simulink model "non_linear_control"  (R2024b)
settings: Solver=FixedStepAuto  StartTime=0.0  StopTime=30  FixedStep=0.01  RelTol=1e-3
settings Model: Creator=olive  LastModifiedBy=olive

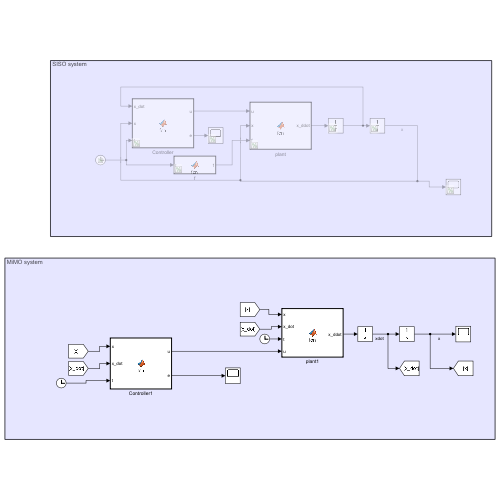
[thumbnail: Simulink's stored preview of the top-level diagram]
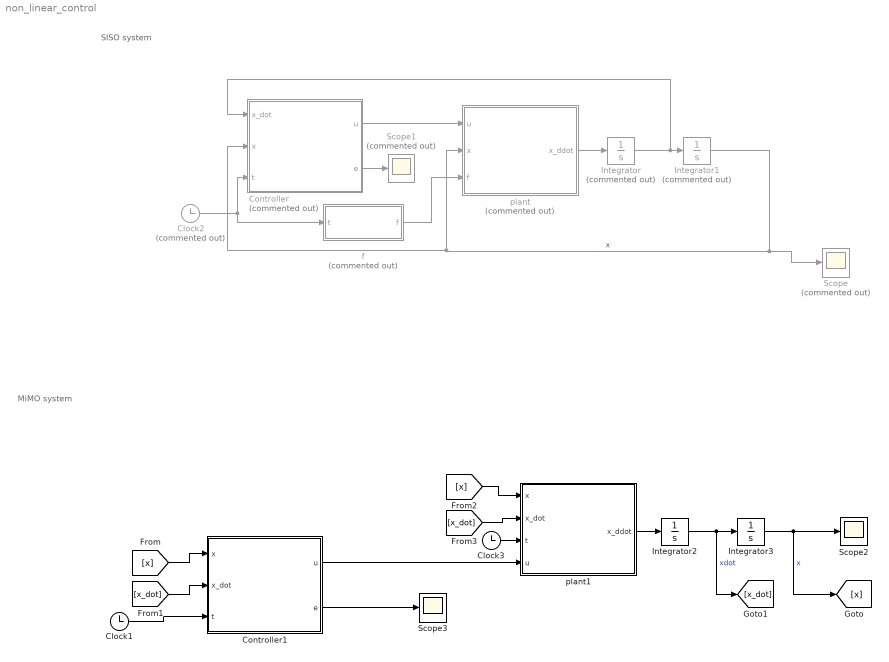
== system non_linear_control ==
  note: MiMO system
  note: SISO system
  Clock1 : Clock
  Clock2 : Clock  Commented=on
  Clock3 : Clock
  Controller : MATLAB Function  Commented=on  TreatAsAtomicUnit=on
  Controller1 : MATLAB Function  TreatAsAtomicUnit=on
  Integrator : Integrator  Commented=on
  Integrator1 : Integrator  Commented=on
  Integrator2 : Integrator  InitialCondition=[0;0]
  Integrator3 : Integrator  InitialCondition=[0;0]
  Scope : Scope  Commented=on
  Scope1 : Scope  Commented=on
  Scope2 : Scope
  Scope3 : Scope
  f : MATLAB Function  Commented=on  TreatAsAtomicUnit=on
  plant : MATLAB Function  Commented=on  TreatAsAtomicUnit=on
  plant1 : MATLAB Function  TreatAsAtomicUnit=on
  wires:
  Controller/1(u) -> plant/1(u)
  f/1(f) -> plant/3(f)
  plant/1(x_ddot) -> Integrator/1
  Integrator/1 -> Controller/1(x_dot), Integrator1/1
  Integrator1/1 -> plant/2(x), Controller/2(x), Scope/1  "x"
  Clock2/1 -> Controller/3(t), f/1(t)
  Controller/2(e) -> Scope1/1
  plant1/1(x_ddot) -> Integrator2/1
  Clock1/1 -> Controller1/3(t)
  Controller1/1(u) -> plant1/4(u)
  Integrator3/1 -> [x], Scope2/1  "x"
  Integrator2/1 -> [x_dot], Integrator3/1  "xdot"
  [x] -> Controller1/1(x)
  Controller1/2(e) -> Scope3/1
  [x_dot] -> Controller1/2(x_dot)
  Clock3/1 -> plant1/3(t)
  [x_dot] -> plant1/2(x_dot)
  [x] -> plant1/1(x)

== matlab function non_linear_control/plant ==
  settings: updateMethod=DISCRETE
  data: u input; x_ddot output; x input; f input
function x_ddot = fcn(u,x,f)
g = 2;
x_ddot = f*x + g*u;
end

== matlab function non_linear_control/f ==
  settings: updateMethod=DISCRETE
  data: f output; t input
function f = fcn(t)
f = sin(t);
end

== matlab function non_linear_control/Controller1 ==
  settings: updateMethod=DISCRETE
  data: x input; u output; x_dot input; t input; e output
function [u,e] = fcn(x,x_dot,t)
%defining f&g
f = [sin(t)*x(1)+cos(t)*x(2);
    10*t*x_dot(1)+sin(t)*sin(t)*x(2)*x_dot(1)];
g = [2 0;
     0 1];
% defining R
r = [10 + sin(0.1*t);
     5 + cos(10*t)];
r_dot = [0.1*cos(0.1*t);
        -10*sin(10*t)];
r_ddot = [-0.01*sin(0.1*t);
          -100*cos(10*t)];
e = x-r;
e_dot = x_dot - r_dot;

kp = 10;
kd = 2;

u = (g^(-1))*(- f - kp*e - kd*e_dot + r_ddot);
end

== matlab function non_linear_control/Controller ==
  settings: updateMethod=DISCRETE
  data: u output; x_dot input; x input; t input; e output
function [u,e] = fcn(x_dot,x,t)
g=2;
f = sin(t)*x;

% defining R
r = 10 + sin(0.1*t);
r_dot = 0.1*cos(0.1*t);
r_ddot = -0.01*sin(0.1*t);
e = x-r;
e_dot = x_dot - r_dot;

kp = 10;
kd = 2;
u = (1/g)*(- f - kp*e - kd*e_dot + r_ddot);
end

== matlab function non_linear_control/plant1 ==
  settings: updateMethod=DISCRETE
  data: x input; x_dot input; t input; u input; x_ddot output
function x_ddot = fcn(x,x_dot,t,u)
f = [sin(t)*x(1)+cos(t)*x(2);
    10*t*x_dot(1)+sin(t)*sin(t)*x(2)*x_dot(1)];

g = [2 0;
     0 1];

x_ddot = f + g*u;
end
